simulink model "vrtut1"  (Simulink 7.4)
settings: Solver=ode45  StartTime=0.0  StopTime=100  RelTol=1e-3
libraries: simulink x3, vrlib x2
Description:
  | Simulink(R) 3D Animation(TM) - Tutorial #1
  | 
  | This model represents a tutorial example, commented in the manual. See the 'Displaying
  | a Virtual World' chapter in the Simulink 3D Animation User's Guide.
settings Model: Creator=Straka  LastModifiedBy=Houska  CovMetricSettings=d  ExtModeTrigMode=oneshot  ExtModeArmWhenConnect=off
settings DataIOCC: LimitDataPoints=off  SignalLoggingName=logsOut
settings OptimizationCC: BlockReduction=off  BooleanDataType=off  InlineInvariantSignals=on  InitFltsAndDblsToZero=on
settings DebuggingCC: CheckExecutionContextPreStartOutputMsg=on  CheckExecutionContextRuntimeOutputMsg=on  SignalResolutionControl=TryResolveAllWithWarning  SolverPrmCheckMsg=none  MultiTaskDSMMsg=warning  MultiTaskCondExecSysMsg=none  StrictBusMsg=None
settings HardwareCC: TargetUnknown=on
settings ModelReferenceCC: UpdateModelReferenceTargets=IfOutOfDate
settings SFSimCC: SimGenerateEmlReport=off
settings RTWCC: IncludeERTFirstTime=on
settings GRTTargetCC: TargetFcnLib=ansi_tfl_tmw.mat

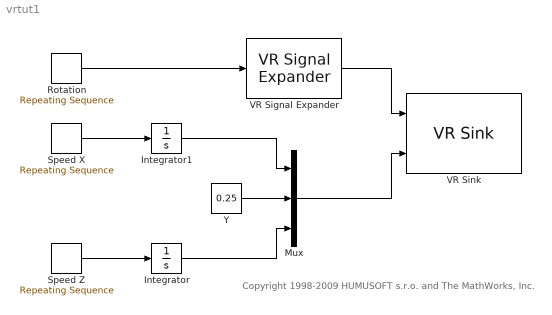
== system vrtut1 ==
  note: Copyright 1998-2009 HUMUSOFT s.r.o. and The MathWorks, Inc.
  Integrator : Integrator  UpperSaturationLimit=Inf  LowerSaturationLimit=-Inf  ZeroCross=off
  Integrator1 : Integrator  InitialCondition=3  UpperSaturationLimit=Inf  LowerSaturationLimit=-Inf  ZeroCross=off
  Mux : Mux  Inputs=3
  Rotation : simulink/Sources/Repeating Sequence  SystemSampleTime=-1  rep_seq_t=[0 20 22 80 82 100]  rep_seq_y=[-1.57 -1.57 -0.7 -0.7 0 0]
  Speed X : simulink/Sources/Repeating Sequence  SystemSampleTime=-1  rep_seq_t=[0 20 22 80 82 100]  rep_seq_y=[0 0 0.33 0.33 0.7 0.7]
  Speed Z : simulink/Sources/Repeating Sequence  SystemSampleTime=-1  rep_seq_t=[0 20 22 80 82 100]  rep_seq_y=[0.55 0.55 0.24 0.24 0 0]
  VR Signal Expander : vrlib/VR Signal Expander  SystemSampleTime=-1  outwidth=4  outidx=4
  VR Sink : vrlib/VR Sink  InstantiateOnLoad=on  SampleTime=0.2  ViewEnable=on  RemoteChange=off  RemoteView=off  FieldsWritten=Automobile.rotation.4.1.double#Automobile.translation.3.1.double  WorldFileName=vrmount.wrl  AutoView=on  VideoDimensions=[]  FigureProperties="{'Position', 'Name', 'Viewpoint', 'CameraBound', 'CameraDirection', 'CameraPosition', 'CameraUpVector', 'ZoomFactor', 'Antialiasing', 'Headlight', 'Lighting', 'NavPanel', 'StatusBar', 'ToolBar', 'Textures', 'Transparency', 'Wireframe', 'NavZones', 'NavMode', 'NavSpeed', 'Record2DCompressMethod', 'Record2DCompressQuality', 'Record2D', 'Record2DFileName', 'Record2DFPS'; [5.0000000000000000e+000  9.2000000000000000e+001  5.7600000000000000e+002  3.8000000000000000e+002], 'VR Car in the Mountains', 'View 1 - Observer', 'on', [0.0000000000000000e+000  0.0000000000000000e+000 -1.0000000000000000e+000], [0.0000000000000000e+000  0.0000000000000000e+000  0.0000000000000000e+000], [0.0000000000000000e+000  1.0000000000000000e+000  0.0000000000000000e+000], [1.0000000000000000e+000], 'off', 'on', 'on', 'halfbar', 'on', 'on', 'on', 'on', 'off', 'off', 'examine', 'normal', 'auto', [7.5000000000000000e+001], 'off', '%f_anim_%n.avi', [1.5000000000000000e+001]}"
  Y : Constant  Value=0.25  OutDataType=sfix(16)  OutScaling=2^0
  wires:
  Speed X/1 -> Integrator1/1
  Speed Z/1 -> Integrator/1
  Y/1 -> Mux/2
  Integrator1/1 -> Mux/1
  Integrator/1 -> Mux/3
  Mux/1 -> VR Sink/2
  VR Signal Expander/1 -> VR Sink/1
  Rotation/1 -> VR Signal Expander/1
